simulink model "FP_DOBS_Delay100_Damping"  (R2016a)
settings: Solver=ode4  StartTime=0.0  StopTime=inf  FixedStep=0.001  RelTol=1e-3
libraries: simulink x3, PhanTorque_3Dof_Library_64Bits x1, sldrtlib x1
settings Model: Creator=Haptic-2  LastModifiedBy=Haptic-2

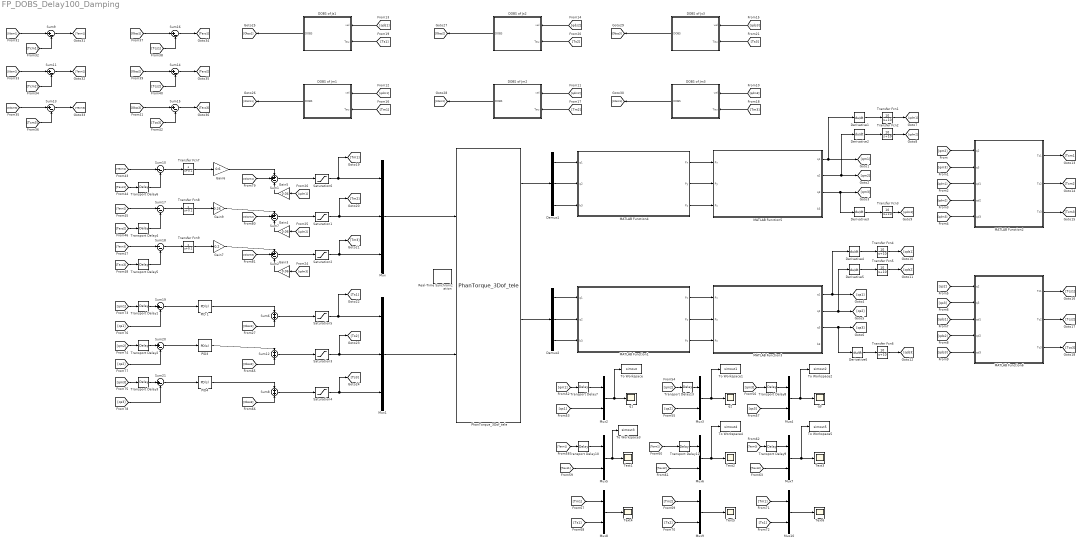
== system FP_DOBS_Delay100_Damping ==
  DOBS of Jm1 : Subsystem
  DOBS of Jm2 : Subsystem
  DOBS of Jm3 : Subsystem
  DOBS of Js1 : Subsystem
  DOBS of Js2 : Subsystem
  DOBS of Js3 : Subsystem
  Demux1 : Demux  Outputs=3
  Demux2 : Demux  Outputs=3
  Derivative{1..6} (6 alike) : Derivative
  Gain3 : Gain  Gain=0.06
  Gain4 : Gain  Gain=0.06
  Gain5 : Gain  Gain=0.04
  Gain6 : Gain  Gain=0.6
  Gain7 : Gain  Gain=0.2
  Gain9 : Gain  Gain=0.26
  MATLAB Function1 : MATLAB Function  TreatAsAtomicUnit=on
  MATLAB Function2 : MATLAB Function  TreatAsAtomicUnit=on
  MATLAB Function3 : MATLAB Function  TreatAsAtomicUnit=on
  MATLAB Function4 : MATLAB Function  TreatAsAtomicUnit=on
  MATLAB Function5 : MATLAB Function  TreatAsAtomicUnit=on
  MATLAB Function6 : MATLAB Function  TreatAsAtomicUnit=on
  Mux : Mux  Inputs=3
  Mux1 : Mux  Inputs=3
  Mux{2..10} (9 alike) : Mux  Inputs=2
  PID 1 : simulink/Continuous/PID Controller  Controller=PD  TimeDomain=Continuous-time  SampleTime=-1  IntegratorMethod=Forward Euler  FilterMethod=Forward Euler  Form=Parallel  UseFilter=on  ControllerParametersSource=internal  P=3  I=0  D=0.1  N=100  InitialConditionSource=internal  InitialConditionForIntegrator=0  InitialConditionForFilter=0  ExternalReset=none  LimitOutput=off  UpperSaturationLimit=inf  LowerSaturationLimit=-inf  LinearizeAsGain=on  AntiWindupMode=none  Kb=1  TrackingMode=off  Kt=1  PParamMin=[]  PParamMax=[]  IParamMin=[]  IParamMax=[]  DParamMin=[]  DParamMax=[]  NParamMin=[]  NParamMax=[]  KbParamMin=[]  KbParamMax=[]  KtParamMin=[]  KtParamMax=[]  POutMin=[]  POutMax=[]  IOutMin=[]  IOutMax=[]  DOutMin=[]  DOutMax=[]  NOutMin=[]  NOutMax=[]  KbOutMin=[]  KbOutMax=[]  KtOutMin=[]  KtOutMax=[]  IntegratorOutMin=[]  IntegratorOutMax=[]  FilterOutMin=[]  FilterOutMax=[]  SumOutMin=[]  SumOutMax=[]  SumI1OutMin=[]  SumI1OutMax=[]  SumI2OutMin=[]  SumI2OutMax=[]  SumI3OutMin=[]  SumI3OutMax=[]  SumDOutMin=[]  SumDOutMax=[]  SaturationOutMin=[]  SaturationOutMax=[]  IntegratorContinuousStateAttributes=''  IntegratorStateMustResolveToSignalObject=off  IntegratorRTWStateStorageClass=Auto  FilterContinuousStateAttributes=''  FilterStateMustResolveToSignalObject=off  FilterRTWStateStorageClass=Auto  DifferentiatorICPrevScaledInput=0  DifferentiatorOutMin=[]  DifferentiatorOutMax=[]
  PID3 : simulink/Continuous/PID Controller  Controller=PD  TimeDomain=Continuous-time  SampleTime=-1  IntegratorMethod=Forward Euler  FilterMethod=Forward Euler  Form=Parallel  UseFilter=on  ControllerParametersSource=internal  P=2.6  I=0  D=0.068  N=100  InitialConditionSource=internal  InitialConditionForIntegrator=0  InitialConditionForFilter=0  ExternalReset=none  LimitOutput=off  UpperSaturationLimit=inf  LowerSaturationLimit=-inf  LinearizeAsGain=on  AntiWindupMode=none  Kb=1  TrackingMode=off  Kt=1  PParamMin=[]  PParamMax=[]  IParamMin=[]  IParamMax=[]  DParamMin=[]  DParamMax=[]  NParamMin=[]  NParamMax=[]  KbParamMin=[]  KbParamMax=[]  KtParamMin=[]  KtParamMax=[]  POutMin=[]  POutMax=[]  IOutMin=[]  IOutMax=[]  DOutMin=[]  DOutMax=[]  NOutMin=[]  NOutMax=[]  KbOutMin=[]  KbOutMax=[]  KtOutMin=[]  KtOutMax=[]  IntegratorOutMin=[]  IntegratorOutMax=[]  FilterOutMin=[]  FilterOutMax=[]  SumOutMin=[]  SumOutMax=[]  SumI1OutMin=[]  SumI1OutMax=[]  SumI2OutMin=[]  SumI2OutMax=[]  SumI3OutMin=[]  SumI3OutMax=[]  SumDOutMin=[]  SumDOutMax=[]  SaturationOutMin=[]  SaturationOutMax=[]  IntegratorContinuousStateAttributes=''  IntegratorStateMustResolveToSignalObject=off  IntegratorRTWStateStorageClass=Auto  FilterContinuousStateAttributes=''  FilterStateMustResolveToSignalObject=off  FilterRTWStateStorageClass=Auto  DifferentiatorICPrevScaledInput=0  DifferentiatorOutMin=[]  DifferentiatorOutMax=[]
  PID4 : simulink/Continuous/PID Controller  Controller=PD  TimeDomain=Continuous-time  SampleTime=-1  IntegratorMethod=Forward Euler  FilterMethod=Forward Euler  Form=Parallel  UseFilter=on  ControllerParametersSource=internal  P=2.926  I=0  D=0.047  N=100  InitialConditionSource=internal  InitialConditionForIntegrator=0  InitialConditionForFilter=0  ExternalReset=none  LimitOutput=off  UpperSaturationLimit=inf  LowerSaturationLimit=-inf  LinearizeAsGain=on  AntiWindupMode=none  Kb=1  TrackingMode=off  Kt=1  PParamMin=[]  PParamMax=[]  IParamMin=[]  IParamMax=[]  DParamMin=[]  DParamMax=[]  NParamMin=[]  NParamMax=[]  KbParamMin=[]  KbParamMax=[]  KtParamMin=[]  KtParamMax=[]  POutMin=[]  POutMax=[]  IOutMin=[]  IOutMax=[]  DOutMin=[]  DOutMax=[]  NOutMin=[]  NOutMax=[]  KbOutMin=[]  KbOutMax=[]  KtOutMin=[]  KtOutMax=[]  IntegratorOutMin=[]  IntegratorOutMax=[]  FilterOutMin=[]  FilterOutMax=[]  SumOutMin=[]  SumOutMax=[]  SumI1OutMin=[]  SumI1OutMax=[]  SumI2OutMin=[]  SumI2OutMax=[]  SumI3OutMin=[]  SumI3OutMax=[]  SumDOutMin=[]  SumDOutMax=[]  SaturationOutMin=[]  SaturationOutMax=[]  IntegratorContinuousStateAttributes=''  IntegratorStateMustResolveToSignalObject=off  IntegratorRTWStateStorageClass=Auto  FilterContinuousStateAttributes=''  FilterStateMustResolveToSignalObject=off  FilterRTWStateStorageClass=Auto  DifferentiatorICPrevScaledInput=0  DifferentiatorOutMin=[]  DifferentiatorOutMax=[]
  PhanTorque_3Dof_tele : PhanTorque_3Dof_Library_64Bits/PhanTorque_3Dof_tele  Haptic1_Name='Left Device'  Haptic2_Name='Right Device'
  Real-Time Synchronization : sldrtlib/Real-Time Synchronization  SampleTime=0.001  MaxMissedTicks=1000  ShowMissedTicks=off  YieldWhenWaiting=off
  Saturation{1..6} (6 alike) : Saturate  UpperLimit=3.5  LowerLimit=-3.5
  Sum1 : Sum  Inputs=++-
  Sum10 : Sum  Inputs=|--
  Sum{9,11,13..16,19..21} (9 alike) : Sum  Inputs=|+-
  Sum12 : Sum
  Sum17 : Sum  Inputs=|--
  Sum18 : Sum  Inputs=|--
  Sum2 : Sum  Inputs=++-
  Sum6 : Sum
  Sum7 : Sum  Inputs=++-
  Sum8 : Sum
  Text{1..6} (6 alike) : Scope
  To Workspace : ToWorkspace  VariableName=simout  SaveFormat=Timeseries  SampleTime=-1
  To Workspace1 : ToWorkspace  VariableName=simout1  SaveFormat=Timeseries  SampleTime=-1
  To Workspace2 : ToWorkspace  VariableName=simout2  SaveFormat=Timeseries  SampleTime=-1
  To Workspace3 : ToWorkspace  VariableName=simout3  SaveFormat=Timeseries  SampleTime=-1
  To Workspace4 : ToWorkspace  VariableName=simout4  SaveFormat=Timeseries  SampleTime=-1
  To Workspace5 : ToWorkspace  VariableName=simout5  SaveFormat=Timeseries  SampleTime=-1
  Transfer Fcn{1..6} (6 alike) : TransferFcn  Numerator=[10]  Denominator=[1 10]
  Transfer Fcn7 : TransferFcn  Numerator=[1 0]  Denominator=[1 0.1]
  Transfer Fcn8 : TransferFcn  Numerator=[1 0]  Denominator=[1 0.1]
  Transfer Fcn9 : TransferFcn  Numerator=[1 0]  Denominator=[1 0.1]
  Transport Delay{1..10,12..13} (12 alike) : TransportDelay  DelayTime=0.1
  q1 : Scope
  q2 : Scope
  q3 : Scope
  wires:
  Mux/1 -> PhanTorque_3Dof_tele/1
  PhanTorque_3Dof_tele/1 -> Demux1/1
  PhanTorque_3Dof_tele/3 -> Demux2/1
  Demux1/1 -> MATLAB Function4/1(q1)
  Demux1/2 -> MATLAB Function4/2(q2)
  Demux1/3 -> MATLAB Function4/3(b3)
  MATLAB Function4/1(Px) -> MATLAB Function5/1(Px)
  MATLAB Function4/2(Py) -> MATLAB Function5/2(Py)
  MATLAB Function4/3(Pz) -> MATLAB Function5/3(Pz)
  Demux2/1 -> MATLAB Function1/1(q1)
  Demux2/2 -> MATLAB Function1/2(q2)
  Demux2/3 -> MATLAB Function1/3(b3)
  MATLAB Function1/1(Px) -> MATLAB Function3/1(Px)
  MATLAB Function1/2(Py) -> MATLAB Function3/2(Py)
  MATLAB Function1/3(Pz) -> MATLAB Function3/3(Pz)
  MATLAB Function5/1(q1) -> Derivative1/1, [qm1]
  MATLAB Function5/2(q2) -> Derivative2/1, [qm2]
  MATLAB Function3/1(q1) -> Derivative4/1, [qs1]
  MATLAB Function3/2(q2) -> Derivative5/1, [qs2]
  MATLAB Function3/3(q3) -> [qs3], Derivative6/1
  [qm2] -> MATLAB Function2/1(q2)
  [qm3] -> MATLAB Function2/2(q3)
  [qdm1] -> MATLAB Function2/3(qd1)
  [qdm2] -> MATLAB Function2/4(qd2)
  [qdm3] -> MATLAB Function2/5(qd3)
  [qs2] -> MATLAB Function6/1(q2)
  [qs3] -> MATLAB Function6/2(q3)
  [qds1] -> MATLAB Function6/3(qd1)
  [qds2] -> MATLAB Function6/4(qd2)
  [qds3] -> MATLAB Function6/5(qd3)
  Derivative1/1 -> Transfer Fcn1/1
  Transfer Fcn1/1 -> [qdm1]
  Derivative2/1 -> Transfer Fcn2/1
  Transfer Fcn2/1 -> [qdm2]
  MATLAB Function5/3(q3) -> Derivative3/1, [qm3]
  Derivative3/1 -> Transfer Fcn3/1
  Transfer Fcn3/1 -> [qdm3]
  Derivative4/1 -> Transfer Fcn4/1
  Derivative5/1 -> Transfer Fcn5/1
  Transfer Fcn4/1 -> [qds1]
  Transfer Fcn5/1 -> [qds2]
  Derivative6/1 -> Transfer Fcn6/1
  Transfer Fcn6/1 -> [qds3]
  MATLAB Function2/1(Tc1) -> [Tcm1]
  MATLAB Function2/2(Tc2) -> [Tcm2]
  MATLAB Function2/3(Tc3) -> [Tcm3]
  MATLAB Function6/1(Tc1) -> [Tcs1]
  MATLAB Function6/2(Tc2) -> [Tcs2]
  MATLAB Function6/3(Tc3) -> [Tcs3]
  [qdm3] -> DOBS of Jm3/1(vel)
  [qds1] -> DOBS of Js1/1(vel)
  [qdm1] -> DOBS of Jm1/1(vel)
  [qdm2] -> DOBS of Jm2/1(vel)
  [qds2] -> DOBS of Js2/1(vel)
  [qds3] -> DOBS of Js3/1(vel)
  Sum1/1 -> Saturation6/1
  Sum7/1 -> Saturation1/1
  Sum2/1 -> Saturation2/1
  Saturation6/1 -> [Tm1], Mux/1
  Saturation1/1 -> Mux/2, [Tm2]
  Saturation2/1 -> Mux/3, [Tm3]
  Sum6/1 -> Saturation5/1
  Sum12/1 -> Saturation3/1
  Sum8/1 -> Saturation4/1
  Saturation5/1 -> Mux1/1, [Ts1]
  Saturation3/1 -> Mux1/2, [Ts2]
  Saturation4/1 -> Mux1/3, [Ts3]
  [Tm1] -> DOBS of Jm1/2(Tau)
  [Tm2] -> DOBS of Jm2/2(Tau)
  [Tm3] -> DOBS of Jm3/2(Tau)
  [Ts1] -> DOBS of Js1/2(Tau)
  [Ts2] -> DOBS of Js2/2(Tau)
  [Ts3] -> DOBS of Js3/2(Tau)
  DOBS of Js1/1(DOBS) -> [Obss1]
  DOBS of Jm1/1(DOBS) -> [Obsm1]
  DOBS of Js2/1(DOBS) -> [Obss2]
  DOBS of Jm2/1(DOBS) -> [Obsm2]
  DOBS of Js3/1(DOBS) -> [Obss3]
  DOBS of Jm3/1(DOBS) -> [Obsm3]
  [Obsm1] -> Sum9/1
  [Tcm1] -> Sum9/2
  [Obsm2] -> Sum11/1
  [Tcm2] -> Sum11/2
  [Obsm3] -> Sum13/1
  [Tcm3] -> Sum13/2
  [Obss1] -> Sum16/1
  [Tcs1] -> Sum16/2
  [Obss2] -> Sum14/1
  [Tcs2] -> Sum14/2
  [Obss3] -> Sum15/1
  [Tcs3] -> Sum15/2
  Sum9/1 -> [Texm1]
  Sum11/1 -> [Texm2]
  Sum13/1 -> [Texm3]
  Sum16/1 -> [Texs1]
  Sum14/1 -> [Texs2]
  Sum15/1 -> [Texs3]
  Mux2/1 -> To Workspace/1, q1/1
  Mux3/1 -> To Workspace1/1, q2/1
  Mux4/1 -> To Workspace2/1, q3/1
  [Texm1] -> Transport Delay10/1
  Mux5/1 -> To Workspace3/1, Text1/1
  [Texm2] -> Transport Delay12/1
  Mux6/1 -> To Workspace4/1, Text2/1
  [Texm3] -> Transport Delay9/1
  Mux7/1 -> To Workspace5/1, Text3/1
  [Tm1] -> Mux8/1
  [Ts1] -> Mux8/2
  Mux8/1 -> Text4/1
  [Tm2] -> Mux9/1
  [Ts2] -> Mux9/2
  Mux9/1 -> Text5/1
  [Tm1] -> Mux10/1
  [Ts1] -> Mux10/2
  Mux10/1 -> Text6/1
  [qm1] -> Transport Delay1/1
  [qm2] -> Transport Delay2/1
  [qm3] -> Transport Delay3/1
  [qs1] -> Sum19/2
  [qs2] -> Sum20/2
  [qs3] -> Sum21/2
  [Texm1] -> Sum10/1
  [Texs1] -> Transport Delay6/1
  [Texm2] -> Sum17/1
  [Texs2] -> Transport Delay4/1
  [Texm3] -> Sum18/1
  [Texs3] -> Transport Delay5/1
  Sum10/1 -> Transfer Fcn7/1
  Sum17/1 -> Transfer Fcn8/1
  Sum18/1 -> Transfer Fcn9/1
  PID 1/1 -> Sum6/1
  PID3/1 -> Sum12/1
  PID4/1 -> Sum8/1
  Mux1/1 -> PhanTorque_3Dof_tele/2
  Sum19/1 -> PID 1/1
  Sum20/1 -> PID3/1
  Sum21/1 -> PID4/1
  Transport Delay1/1 -> Sum19/1
  Transport Delay3/1 -> Sum21/1
  Transport Delay2/1 -> Sum20/1
  Transport Delay5/1 -> Sum18/2
  Transport Delay4/1 -> Sum17/2
  Transport Delay6/1 -> Sum10/2
  Gain3/1 -> Sum2/3
  [qdm3] -> Gain3/1
  Gain4/1 -> Sum7/3
  [qdm2] -> Gain4/1
  Gain5/1 -> Sum1/3
  [qdm1] -> Gain5/1
  [Obss3] -> Sum8/2
  [Obss2] -> Sum12/2
  [Obss1] -> Sum6/2
  [Obsm1] -> Sum1/2
  [Obsm2] -> Sum7/2
  [Obsm3] -> Sum2/2
  Gain6/1 -> Sum1/1
  Gain9/1 -> Sum7/1
  Gain7/1 -> Sum2/1
  [qm1] -> Transport Delay7/1
  [qm2] -> Transport Delay13/1
  [qm3] -> Transport Delay8/1
  [qs2] -> Mux3/2
  [qs3] -> Mux4/2
  [Texs3] -> Mux7/2
  [Texs2] -> Mux6/2
  [Texs1] -> Mux5/2
  Transport Delay13/1 -> Mux3/1
  Transport Delay8/1 -> Mux4/1
  Transport Delay9/1 -> Mux7/1
  Transport Delay10/1 -> Mux5/1
  Transport Delay12/1 -> Mux6/1
  Transfer Fcn7/1 -> Gain6/1
  Transfer Fcn8/1 -> Gain9/1
  Transfer Fcn9/1 -> Gain7/1
  Transport Delay7/1 -> Mux2/1
  [qs1] -> Mux2/2

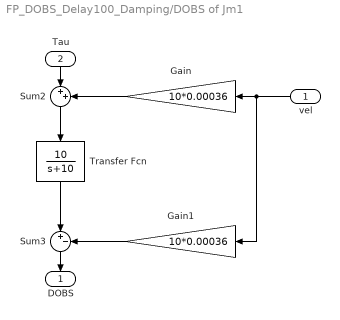
== system FP_DOBS_Delay100_Damping/DOBS of Jm1 ==
  vel : Inport
  Tau : Inport  Port=2
  Gain : Gain  Gain=10*0.00036
  Gain1 : Gain  Gain=10*0.00036
  Sum2 : Sum  Inputs=|++
  Sum3 : Sum  Inputs=|+-
  Transfer Fcn : TransferFcn  Numerator=[10]  Denominator=[1 10]
  DOBS : Outport
  wires:
  Gain/1 -> Sum2/2
  Sum2/1 -> Transfer Fcn/1
  Transfer Fcn/1 -> Sum3/1
  Gain1/1 -> Sum3/2
  Tau/1 -> Sum2/1
  Sum3/1 -> DOBS/1
  vel/1 -> Gain1/1, Gain/1

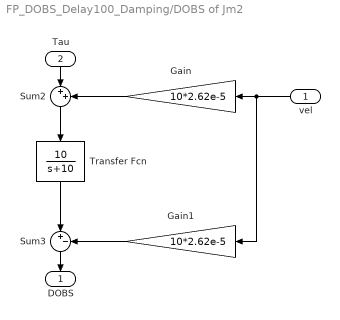
== system FP_DOBS_Delay100_Damping/DOBS of Jm2 ==
  vel : Inport
  Tau : Inport  Port=2
  Gain : Gain  Gain=10*2.62e-5
  Gain1 : Gain  Gain=10*2.62e-5
  Sum2 : Sum  Inputs=|++
  Sum3 : Sum  Inputs=|+-
  Transfer Fcn : TransferFcn  Numerator=[10]  Denominator=[1 10]
  DOBS : Outport
  wires:
  vel/1 -> Gain1/1, Gain/1
  Sum3/1 -> DOBS/1
  Tau/1 -> Sum2/1
  Gain1/1 -> Sum3/2
  Transfer Fcn/1 -> Sum3/1
  Sum2/1 -> Transfer Fcn/1
  Gain/1 -> Sum2/2

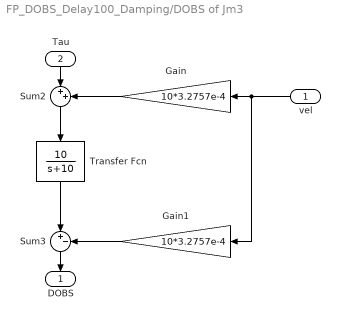
== system FP_DOBS_Delay100_Damping/DOBS of Jm3 ==
  vel : Inport
  Tau : Inport  Port=2
  Gain : Gain  Gain=10*3.2757e-4
  Gain1 : Gain  Gain=10*3.2757e-4
  Sum2 : Sum  Inputs=|++
  Sum3 : Sum  Inputs=|+-
  Transfer Fcn : TransferFcn  Numerator=[10]  Denominator=[1 10]
  DOBS : Outport
  wires:
  Gain/1 -> Sum2/2
  Sum2/1 -> Transfer Fcn/1
  Transfer Fcn/1 -> Sum3/1
  Gain1/1 -> Sum3/2
  Tau/1 -> Sum2/1
  Sum3/1 -> DOBS/1
  vel/1 -> Gain1/1, Gain/1

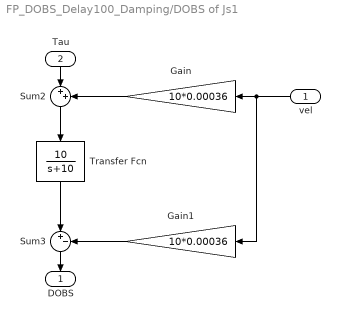
== system FP_DOBS_Delay100_Damping/DOBS of Js1 ==
  vel : Inport
  Tau : Inport  Port=2
  Gain : Gain  Gain=10*0.00036
  Gain1 : Gain  Gain=10*0.00036
  Sum2 : Sum  Inputs=|++
  Sum3 : Sum  Inputs=|+-
  Transfer Fcn : TransferFcn  Numerator=[10]  Denominator=[1 10]
  DOBS : Outport
  wires:
  vel/1 -> Gain/1, Gain1/1
  Sum3/1 -> DOBS/1
  Tau/1 -> Sum2/1
  Gain1/1 -> Sum3/2
  Transfer Fcn/1 -> Sum3/1
  Sum2/1 -> Transfer Fcn/1
  Gain/1 -> Sum2/2

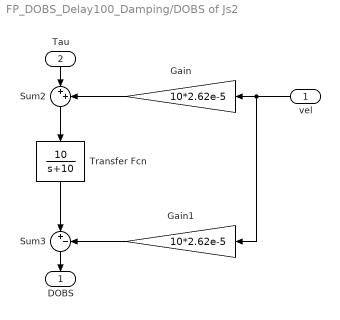
== system FP_DOBS_Delay100_Damping/DOBS of Js2 ==
  vel : Inport
  Tau : Inport  Port=2
  Gain : Gain  Gain=10*2.62e-5
  Gain1 : Gain  Gain=10*2.62e-5
  Sum2 : Sum  Inputs=|++
  Sum3 : Sum  Inputs=|+-
  Transfer Fcn : TransferFcn  Numerator=[10]  Denominator=[1 10]
  DOBS : Outport
  wires:
  Gain/1 -> Sum2/2
  Sum2/1 -> Transfer Fcn/1
  Transfer Fcn/1 -> Sum3/1
  Gain1/1 -> Sum3/2
  Tau/1 -> Sum2/1
  Sum3/1 -> DOBS/1
  vel/1 -> Gain/1, Gain1/1

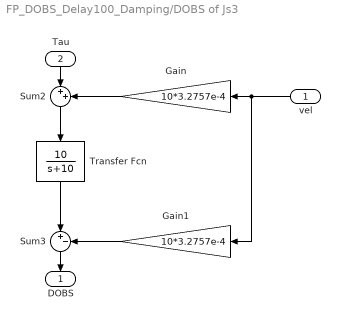
== system FP_DOBS_Delay100_Damping/DOBS of Js3 ==
  vel : Inport
  Tau : Inport  Port=2
  Gain : Gain  Gain=10*3.2757e-4
  Gain1 : Gain  Gain=10*3.2757e-4
  Sum2 : Sum  Inputs=|++
  Sum3 : Sum  Inputs=|+-
  Transfer Fcn : TransferFcn  Numerator=[10]  Denominator=[1 10]
  DOBS : Outport
  wires:
  vel/1 -> Gain/1, Gain1/1
  Sum3/1 -> DOBS/1
  Tau/1 -> Sum2/1
  Gain1/1 -> Sum3/2
  Transfer Fcn/1 -> Sum3/1
  Sum2/1 -> Transfer Fcn/1
  Gain/1 -> Sum2/2

== matlab function FP_DOBS_Delay100_Damping/MATLAB Function1 ==
  data: q1 input; Px output; q2 input; b3 input; Py output; Pz output
function [Px, Py, Pz] = fcn(q1,q2,b3)
%#codegen
% q4=0;
% a3=0.133;
% d1=0.170;
% d4=0.133;
% q3=b3+3*pi/2;
% Tw=[0 1 0 0;1 0 0 0;0 0 1 0;0 0 0 1]; %denote translation
% T01=[cos(q1) -sin(q1) 0 0; sin(q1) cos(q1) 0 0; 0 0 1 d1; 0 0 0 1];
% T12=[cos(q2) -sin(q2) 0 0; 0 0 -1 0; sin(q2) cos(q2) 0 0; 0 0 0 1];
% T23=[cos(q3) -sin(q3) 0 a3; sin(q3) cos(q3) 0 0; 0 0 1 0; 0 0 0 1];
% T34=[cos(q4) -sin(q4) 0 d4; sin(q4) cos(q4) 0 0; 0 0 1 0; 0 0 0 1];
% T04=Tw*T01*T12*T23*T34;
% %simplify(T04)
% P=T04(1:3,4);
% Px=P(1);
% Py=P(2);
% Pz=P(3);

q4=0;
a3=0.133;
d1=0.170;
d4=0.133;
q3=3*pi/2-q2+b3;
Tw=[0 1 0 0;1 0 0 0;0 0 1 0;0 0 0 1]; %denote translation
T01=[cos(q1) -sin(q1) 0 0; sin(q1) cos(q1) 0 0; 0 0 1 d1; 0 0 0 1];
T12=[cos(q2) -sin(q2) 0 0; 0 0 -1 0; sin(q2) cos(q2) 0 0; 0 0 0 1];
T23=[cos(q3) -sin(q3) 0 a3; sin(q3) cos(q3) 0 0; 0 0 1 0; 0 0 0 1];
T34=[cos(q4) -sin(q4) 0 d4; sin(q4) cos(q4) 0 0;0 0 1 0; 0 0 0 1];
T04=Tw*T01*T12*T23*T34;
%simplify(T04)
P=T04(1:3,4);
Px=P(1);
Py=P(2);
Pz=P(3);

== matlab function FP_DOBS_Delay100_Damping/MATLAB Function3 ==
  data: Px input; q1 output; Py input; Pz input; q2 output; q3 output; b3 output
function [q1,q2,q3,b3] = fcn(Px,Py,Pz)
%#codegen
a3=0.133;
d1=0.170;
d4=0.133;
q1=atan2(Px,Py);
h=sqrt((Px^2)+(Py^2)+((Pz-d1)^2));
R=sqrt(Px^2+Py^2);
alfa=acos(((a3^2+d4^2)-h^2)/(2*a3*d4));
beta=acos(((a3^2+h^2)-d4^2)/(2*a3*h));
fi=atan2((Pz-d1),R);
q2=beta+fi;
q3=alfa+pi;
b3=q3-(3*pi/2)+q2;

== matlab function FP_DOBS_Delay100_Damping/MATLAB Function2 ==
  data: Tc1 output; Tc2 output; q2 input; q3 input; qd1 input; qd2 input; Tc3 output; qd3 input
function [Tc1,Tc2,Tc3] = fcn(q2,q3,qd1,qd2,qd3)
m2=0.04;
m3=0.08;
a3=0.133;
d4=0.133;
g=9.81;
l2=a3/3;
l3=5*d4/6;

C=[-2*m2*l2^2*sin(q2)*qd1*qd2-2*m3*a3^2*sin(q2)*qd1*qd2-2*m3*a3*l3*sin(q2)*cos(q2+q3)*qd1*qd2-2*m3*a3*l3*cos(q2)*sin(q2+q3)*qd1*(qd2+qd3)-2*m3*a3*l3*sin(q2+q3)*qd1*(qd2+qd3);
    -2*m3*a3*l3*sin(q3)*qd2*qd3-m3*a3*l3*sin(q3)*qd3^2+0.5*m2*l2^2*sin(2*q2)*qd1^2+0.5*m3*a3^2*sin(2*q2)*qd1^2+m3*a3*l3*sin(2*q2+2*q3)*qd1^2+0.5*m3*l3^2*sin(2*q2+2*q3)*qd1^2;
    -m3*a3*l3*sin(q3)*qd2*qd3+0.5*m3*a3*l3*sin(q3)*qd1^2+m3*a3*l3*sin(q3)*qd2^2+m3*a3*l3*sin(q3)*qd2*qd3+0.5*m3*a3*l3*sin(2*q2+q3)*qd1^2+0.5*m3*l3^2*sin(2*q2+2*q3)*qd1^2];
G=[ 0;
    (m2+m3)*l2*g*cos(q2)+m3*g*l3*cos(q2+q3);
     m3*g*l3*cos(q2+q3)];

Tc1=C(1,1)+G(1,1);
Tc2=C(2,1)+G(2,1);
Tc3=C(3,1)+G(3,1);

== matlab function FP_DOBS_Delay100_Damping/MATLAB Function6 ==
  data: Tc1 output; Tc2 output; q2 input; q3 input; qd1 input; qd2 input; Tc3 output; qd3 input
function [Tc1,Tc2,Tc3] = fcn(q2,q3,qd1,qd2,qd3)
m2=0.04;
m3=0.08;
a3=0.133;
d4=0.133;
g=9.81;
l2=a3/3;
l3=5*d4/6;

C=[-2*m2*l2^2*sin(q2)*qd1*qd2-2*m3*a3^2*sin(q2)*qd1*qd2-2*m3*a3*l3*sin(q2)*cos(q2+q3)*qd1*qd2-2*m3*a3*l3*cos(q2)*sin(q2+q3)*qd1*(qd2+qd3)-2*m3*a3*l3*sin(q2+q3)*qd1*(qd2+qd3);
    -2*m3*a3*l3*sin(q3)*qd2*qd3-m3*a3*l3*sin(q3)*qd3^2+0.5*m2*l2^2*sin(2*q2)*qd1^2+0.5*m3*a3^2*sin(2*q2)*qd1^2+m3*a3*l3*sin(2*q2+2*q3)*qd1^2+0.5*m3*l3^2*sin(2*q2+2*q3)*qd1^2;
    -m3*a3*l3*sin(q3)*qd2*qd3+0.5*m3*a3*l3*sin(q3)*qd1^2+m3*a3*l3*sin(q3)*qd2^2+m3*a3*l3*sin(q3)*qd2*qd3+0.5*m3*a3*l3*sin(2*q2+q3)*qd1^2+0.5*m3*l3^2*sin(2*q2+2*q3)*qd1^2];
G=[ 0;
    (m2+m3)*l2*g*cos(q2)+m3*g*l3*cos(q2+q3);
     m3*g*l3*cos(q2+q3)];

Tc1=C(1,1)+G(1,1);
Tc2=C(2,1)+G(2,1);
Tc3=C(3,1)+G(3,1);

== matlab function FP_DOBS_Delay100_Damping/MATLAB Function4 ==
  data: q1 input; Px output; q2 input; b3 input; Py output; Pz output
function [Px, Py, Pz] = fcn(q1,q2,b3)
%#codegen
% q4=0;
% a3=0.133;
% d1=0.170;
% d4=0.133;
% q3=b3+3*pi/2;
% Tw=[0 1 0 0;1 0 0 0;0 0 1 0;0 0 0 1]; %denote translation
% T01=[cos(q1) -sin(q1) 0 0; sin(q1) cos(q1) 0 0; 0 0 1 d1; 0 0 0 1];
% T12=[cos(q2) -sin(q2) 0 0; 0 0 -1 0; sin(q2) cos(q2) 0 0; 0 0 0 1];
% T23=[cos(q3) -sin(q3) 0 a3; sin(q3) cos(q3) 0 0; 0 0 1 0; 0 0 0 1];
% T34=[cos(q4) -sin(q4) 0 d4; sin(q4) cos(q4) 0 0; 0 0 1 0; 0 0 0 1];
% T04=Tw*T01*T12*T23*T34;
% %simplify(T04)
% P=T04(1:3,4);
% Px=P(1);
% Py=P(2);
% Pz=P(3);

q4=0;
a3=0.133;
d1=0.170;
d4=0.133;
q3=3*pi/2-q2+b3;
Tw=[0 1 0 0;1 0 0 0;0 0 1 0;0 0 0 1]; %denote translation
T01=[cos(q1) -sin(q1) 0 0; sin(q1) cos(q1) 0 0; 0 0 1 d1; 0 0 0 1];
T12=[cos(q2) -sin(q2) 0 0; 0 0 -1 0; sin(q2) cos(q2) 0 0; 0 0 0 1];
T23=[cos(q3) -sin(q3) 0 a3; sin(q3) cos(q3) 0 0; 0 0 1 0; 0 0 0 1];
T34=[cos(q4) -sin(q4) 0 d4; sin(q4) cos(q4) 0 0;0 0 1 0; 0 0 0 1];
T04=Tw*T01*T12*T23*T34;
%simplify(T04)
P=T04(1:3,4);
Px=P(1);
Py=P(2);
Pz=P(3);

== matlab function FP_DOBS_Delay100_Damping/MATLAB Function5 ==
  data: Px input; q1 output; Py input; Pz input; q2 output; q3 output; b3 output
function [q1,q2,q3,b3] = fcn(Px,Py,Pz)
%#codegen
a3=0.133;
d1=0.170;
d4=0.133;
q1=atan2(Px,Py);
h=sqrt((Px^2)+(Py^2)+((Pz-d1)^2));
R=sqrt(Px^2+Py^2);
alfa=acos(((a3^2+d4^2)-h^2)/(2*a3*d4));
beta=acos(((a3^2+h^2)-d4^2)/(2*a3*h));
fi=atan2((Pz-d1),R);
q2=beta+fi;
q3=alfa+pi;
b3=q3-(3*pi/2)+q2;
